simulink model "Simulation_model_full"  (R2021a)
settings: Solver=ode23t  StartTime=0.0  StopTime=6  FixedStep=T  RelTol=1e-3
values from neighbouring files (symbols this model uses):
  C_dc = Cb*c_dc_pu    [parameters.m]
  C_f = Cb*c_f_pu    [parameters.m]
  f_SM = fb    (= 50)    [parameters.m]
  fb = 50    [parameters.m]
  ff_SM = 0.01322    [parameters.m]
  Ib = 2/3*Sb/Vb    [parameters.m]
  Ib_dc = Sb/Vb_dc    [parameters.m]
  ic_SM = 0.8    [parameters.m]
  K_ad = 1.5    [parameters.m]
  K_ffv = 0    [parameters.m]
  K_ic = K_pc/T_1    [parameters.m]
  K_idc = K_pdc/T_idc    (= 250)    [parameters.m]
  K_iPLL = a^2*T_fPLL    (= 0.09)    [parameters.m]
  K_iv = K_pv/T_iv    (= 92.0050761421)    [parameters.m]
  K_iv_SM = K_pv_SM/T_iv_SM    (= 70)    [parameters.m]
  K_omega = 20    [parameters.m]
  K_omega_SM = 40    [parameters.m]
  K_pc = l_f_pu/(4*pi*fb*T_sum)    (= 1.27323954474)    [parameters.m]
  K_pdc = 25    [parameters.m]
  K_pPLL = 1/(a*2*pi*T_fPLL)    (= 5.30516476973)    [parameters.m]
  K_pv = 0.29    [parameters.m]
  K_pv_SM = 35    [parameters.m]
  K_vco = 2*pi    (= 6.28318530718)    [parameters.m]
  Kd = 40    [parameters.m]
  Kq = 0.1    [parameters.m]
  Kq_SM = 0.1    [parameters.m]
  L_f = Lb*l_f_pu    [parameters.m]
  l_f_pu = 0.08    [parameters.m]
  lfd_SM = 0.531    [parameters.m]
  llkd = 2.655    [parameters.m]
  llkq1 = 0.2408    [parameters.m]
  lls_SM = 0.08    [parameters.m]
  lmd_SM = 2.81    [parameters.m]
  lmq_SM = 1.64    [parameters.m]
  omega_ad = 50    [parameters.m]
  omega_b = 2*pi*fb    (= 314.159265359)    [parameters.m]
  omega_d = 5    [parameters.m]
  omega_qf = 200    [parameters.m]
  omega_qf_SM = 200    [parameters.m]
  omega_vf = 200    [parameters.m]
  p_h = 0.1    [parameters.m]
  pp_SM = 2    [parameters.m]
  R_lf = Rb*r_lf_pu    [parameters.m]
  rfd_SM = 0.004319    [parameters.m]
  rkd = 0.2343    [parameters.m]
  rkq1 = 0.03365    [parameters.m]
  rs_SM = 0.01524    [parameters.m]
  S_SM = Sb    (= 1000000)    [parameters.m]
  Sb = 1e6    (= 1000000)    [parameters.m]
  T = 1e-4    (= 0.0001)    [parameters.m]
  T_fPLL = 10e-3    (= 0.01)    [parameters.m]
  T_gt_SM = 0.5    [parameters.m]
  Ta = 4    [parameters.m]
  V_dc_bat = 1200    [parameters.m]
  v_dc_ref = 1    [parameters.m]
  V_SM = V    (= 690)    [parameters.m]
  Vb = V*sqrt(2)/sqrt(3)    [parameters.m]
  Vb_dc = Vb*2    [parameters.m]
undefined symbols (not defined in the file or in its folder): D1, Delta
libraries: simulink_extras x36, spsDiodeLib x24, spsThreePhaseVIMeasurementLib x16, spsThreePhaseSeriesRLCBranchLib x14, spsPower3phInstantaneousLib x8, spsVoltageMeasurementLib x5, spsControlledCurrentSourceLib x4, spsUniversalBridgeLib x4, spsParallelRLCBranchLib x2, spsSeriesRLCBranchLib x2, spsSynchronousMachinepuFundamentalLib x2, spsThreePhaseParallelRLCLoadLib x2
(part 2 of 3)

== system Simulation_model_full/Automatic Voltage Regulator SM A ==
  v_hat* : Inport
  v_hat_o : Inport  Port=2
  q* : Inport  Port=3
  qo : Inport  Port=4
  Gain15 : Gain  Gain=K_iv_SM
  Gain2 : Gain  Gain=Kq_SM
  Gain8 : Gain  Gain=K_pv_SM
  Integrator : Integrator
  Sum1 : Sum  Inputs=-++
  Sum2 : Sum  Inputs=|+-
  Sum9 : Sum  Inputs=|++
  Transfer Fcn (with initial outputs) : simulink_extras/Additional Linear/Transfer Fcn (with initial outputs)  N=[omega_qf_SM]  D="[1  omega_qf_SM]"  Y0=0  U0=0
  v_hat_e : Outport
  wires:
  Integrator/1 -> Sum9/2
  Sum1/1 -> Gain15/1, Gain8/1
  Gain15/1 -> Integrator/1
  Gain8/1 -> Sum9/1
  q*/1 -> Sum2/1
  qo/1 -> Transfer Fcn (with initial outputs)/1
  Transfer Fcn (with initial outputs)/1 -> Sum2/2
  Sum2/1 -> Gain2/1
  v_hat*/1 -> Sum1/2
  Gain2/1 -> Sum1/3
  Sum9/1 -> v_hat_e/1
  v_hat_o/1 -> Sum1/1

== system Simulation_model_full/Automatic Voltage Regulator SM B ==
  v_hat* : Inport
  v_hat_o : Inport  Port=2
  q* : Inport  Port=3
  qo : Inport  Port=4
  Gain15 : Gain  Gain=K_iv_SM
  Gain2 : Gain  Gain=Kq_SM
  Gain8 : Gain  Gain=K_pv_SM
  Integrator : Integrator
  Sum1 : Sum  Inputs=-++
  Sum2 : Sum  Inputs=|+-
  Sum9 : Sum  Inputs=|++
  Transfer Fcn (with initial outputs) : simulink_extras/Additional Linear/Transfer Fcn (with initial outputs)  N=[omega_qf_SM]  D="[1  omega_qf_SM]"  Y0=0  U0=0
  v_hat_e : Outport
  wires:
  Integrator/1 -> Sum9/2
  Sum1/1 -> Gain15/1, Gain8/1
  Gain15/1 -> Integrator/1
  Gain8/1 -> Sum9/1
  q*/1 -> Sum2/1
  qo/1 -> Transfer Fcn (with initial outputs)/1
  Transfer Fcn (with initial outputs)/1 -> Sum2/2
  Sum2/1 -> Gain2/1
  v_hat*/1 -> Sum1/2
  Gain2/1 -> Sum1/3
  Sum9/1 -> v_hat_e/1
  v_hat_o/1 -> Sum1/1

== system Simulation_model_full/Diesel Generator Governor Model SM A ==
  p*_sm : Inport
  omega_sm* : Inport  Port=2
  omega_sm : Inport  Port=3
  Sum1 : Sum  Inputs=++|
  Sum2 : Sum  Inputs=|+-
  Transfer Fcn (with initial outputs)2 : simulink_extras/Additional Linear/Transfer Fcn (with initial outputs)  N=[1]  D=[T_gt_SM 1]  Y0=0  U0=0
  "k_omega, sm" : Gain  Gain=K_omega_SM
  tau_dg : Outport
  wires:
  omega_sm*/1 -> Sum2/1
  omega_sm/1 -> Sum2/2
  Sum2/1 -> "k_omega, sm"/1
  "k_omega, sm"/1 -> Sum1/2
  p*_sm/1 -> Sum1/1
  Sum1/1 -> Transfer Fcn (with initial outputs)2/1
  Transfer Fcn (with initial outputs)2/1 -> tau_dg/1

== system Simulation_model_full/Diesel Generator Governor Model SM B ==
  p*_sm : Inport
  omega_sm* : Inport  Port=2
  omega_sm : Inport  Port=3
  Sum1 : Sum  Inputs=++|
  Sum2 : Sum  Inputs=|+-
  Transfer Fcn (with initial outputs)2 : simulink_extras/Additional Linear/Transfer Fcn (with initial outputs)  N=[1]  D=[T_gt_SM 1]  Y0=0  U0=0
  "k_omega, sm" : Gain  Gain=K_omega_SM
  tau_dg : Outport
  wires:
  omega_sm*/1 -> Sum2/1
  omega_sm/1 -> Sum2/2
  Sum2/1 -> "k_omega, sm"/1
  "k_omega, sm"/1 -> Sum1/2
  p*_sm/1 -> Sum1/1
  Sum1/1 -> Transfer Fcn (with initial outputs)2/1
  Transfer Fcn (with initial outputs)2/1 -> tau_dg/1

== system Simulation_model_full/P to I VSC A ==
  p_load : Inport
  v_dc : Inport  Port=2
  Divide : Product  Inputs=*/
  Saturation : Saturate  UpperLimit=1.5  LowerLimit=0.5
  Transfer Fcn (with initial outputs) : simulink_extras/Additional Linear/Transfer Fcn (with initial outputs)  N=[200]  D="[1  200]"  Y0=1  U0=1
  i_dc : Outport
  Out2 : Outport  Port=2
  wires:
  Divide/1 -> i_dc/1
  v_dc/1 -> Saturation/1
  Saturation/1 -> Transfer Fcn (with initial outputs)/1
  p_load/1 -> Divide/1
  Transfer Fcn (with initial outputs)/1 -> Divide/2

== system Simulation_model_full/P to I VSC B ==
  p_load : Inport
  v_dc : Inport  Port=2
  Divide : Product  Inputs=*/
  Saturation : Saturate  UpperLimit=1.5  LowerLimit=0.5
  Transfer Fcn (with initial outputs) : simulink_extras/Additional Linear/Transfer Fcn (with initial outputs)  N=[200]  D="[1  200]"  Y0=1  U0=1
  i_dc : Outport
  wires:
  Divide/1 -> i_dc/1
  v_dc/1 -> Saturation/1
  Saturation/1 -> Transfer Fcn (with initial outputs)/1
  p_load/1 -> Divide/1
  Transfer Fcn (with initial outputs)/1 -> Divide/2

== system Simulation_model_full/P to I 12puls A ==
  p* : Inport
  v_dc : Inport  Port=2
  Divide : Product  Inputs=*/
  Saturation : Saturate  UpperLimit=1.5  LowerLimit=0.5
  Transfer Fcn (with initial outputs) : simulink_extras/Additional Linear/Transfer Fcn (with initial outputs)  N=[200]  D="[1  200]"  Y0=1  U0=1
  i_dc : Outport
  wires:
  Divide/1 -> i_dc/1
  v_dc/1 -> Saturation/1
  Saturation/1 -> Transfer Fcn (with initial outputs)/1
  p*/1 -> Divide/1
  Transfer Fcn (with initial outputs)/1 -> Divide/2

== system Simulation_model_full/P to I 12puls B ==
  p* : Inport
  v_dc : Inport  Port=2
  Divide : Product  Inputs=*/
  Saturation : Saturate  UpperLimit=1.5  LowerLimit=0.5
  Transfer Fcn (with initial outputs) : simulink_extras/Additional Linear/Transfer Fcn (with initial outputs)  N=[200]  D="[1  200]"  Y0=1  U0=1
  i_dc : Outport
  wires:
  Divide/1 -> i_dc/1
  v_dc/1 -> Saturation/1
  Saturation/1 -> Transfer Fcn (with initial outputs)/1
  p*/1 -> Divide/1
  Transfer Fcn (with initial outputs)/1 -> Divide/2

== system Simulation_model_full/PLL grid ==
  Vo : Inport
  Atan2 : Trigonometry  Operator=atan2  OutputSignalType=real
  Constant1 : Constant  Value=fb
  Demux : Demux  Outputs=3
  Gain : Gain  Gain=K_vco
  Gain12 : Gain  Gain=1/omega_b
  Gain17 : Gain  Gain=K_iPLL
  Gain18 : Gain  Gain=K_pPLL
  Integrator2 : Integrator
  Park : MATLAB Function  TreatAsAtomicUnit=on
  Sum1 : Sum  Inputs=++|
  Sum10 : Sum  Inputs=++|
  Terminator : Terminator
  Transfer Fcn (with initial outputs)1 : simulink_extras/Additional Linear/Transfer Fcn (with initial outputs)  N=[1]  D=[T_fPLL, 1]  Y0=0  U0=0
  Transfer Fcn (with initial outputs)3 : simulink_extras/Additional Linear/Transfer Fcn (with initial outputs)  N=[1]  D=[T_fPLL, 1]  Y0=1  U0=1
  VCO : Integrator  WrapState=on  WrappedStateUpperValue=2*pi  WrappedStateLowerValue=0
  abs vhat_f VSM : MATLAB Function  TreatAsAtomicUnit=on
  omega : Outport
  v_hat : Outport  Port=2
  wires:
  Transfer Fcn (with initial outputs)1/1 -> Atan2/1, abs vhat_f VSM/2(vq)
  Transfer Fcn (with initial outputs)3/1 -> Atan2/2, abs vhat_f VSM/1(vd)
  VCO/1 -> Park/1(theta)
  Sum1/1 -> Gain/1
  Gain/1 -> Gain12/1, VCO/1
  Constant1/1 -> Sum1/1
  Park/1(dq0) -> Demux/1
  Sum10/1 -> Sum1/2
  Atan2/1 -> Gain18/1, Gain17/1
  Demux/1 -> Transfer Fcn (with initial outputs)3/1
  Demux/2 -> Transfer Fcn (with initial outputs)1/1
  Vo/1 -> Park/2(abc)
  Gain18/1 -> Sum10/2
  Integrator2/1 -> Sum10/1
  Gain17/1 -> Integrator2/1
  Gain12/1 -> omega/1
  Demux/3 -> Terminator/1
  abs vhat_f VSM/1(v_abs) -> v_hat/1

== system Simulation_model_full/PLL grid1 ==
  Vo : Inport
  Atan2 : Trigonometry  Operator=atan2  OutputSignalType=real
  Constant1 : Constant  Value=fb
  Demux : Demux  Outputs=3
  Gain : Gain  Gain=K_vco
  Gain12 : Gain  Gain=1/omega_b
  Gain17 : Gain  Gain=K_iPLL
  Gain18 : Gain  Gain=K_pPLL
  Integrator2 : Integrator
  Park : MATLAB Function  TreatAsAtomicUnit=on
  Sum1 : Sum  Inputs=++|
  Sum10 : Sum  Inputs=++|
  Terminator : Terminator
  Transfer Fcn (with initial outputs)1 : simulink_extras/Additional Linear/Transfer Fcn (with initial outputs)  N=[1]  D=[T_fPLL, 1]  Y0=0  U0=0
  Transfer Fcn (with initial outputs)3 : simulink_extras/Additional Linear/Transfer Fcn (with initial outputs)  N=[1]  D=[T_fPLL, 1]  Y0=1  U0=1
  VCO : Integrator  WrapState=on  WrappedStateUpperValue=2*pi  WrappedStateLowerValue=0
  abs vhat_f VSM : MATLAB Function  TreatAsAtomicUnit=on
  omega : Outport
  v_hat : Outport  Port=2
  wires:
  Transfer Fcn (with initial outputs)1/1 -> Atan2/1, abs vhat_f VSM/2(vq)
  Transfer Fcn (with initial outputs)3/1 -> Atan2/2, abs vhat_f VSM/1(vd)
  VCO/1 -> Park/1(theta)
  Sum1/1 -> Gain/1
  Gain/1 -> Gain12/1, VCO/1
  Constant1/1 -> Sum1/1
  Park/1(dq0) -> Demux/1
  Sum10/1 -> Sum1/2
  Atan2/1 -> Gain18/1, Gain17/1
  Demux/1 -> Transfer Fcn (with initial outputs)3/1
  Demux/2 -> Transfer Fcn (with initial outputs)1/1
  Vo/1 -> Park/2(abc)
  Gain18/1 -> Sum10/2
  Integrator2/1 -> Sum10/1
  Gain17/1 -> Integrator2/1
  Gain12/1 -> omega/1
  Demux/3 -> Terminator/1
  abs vhat_f VSM/1(v_abs) -> v_hat/1

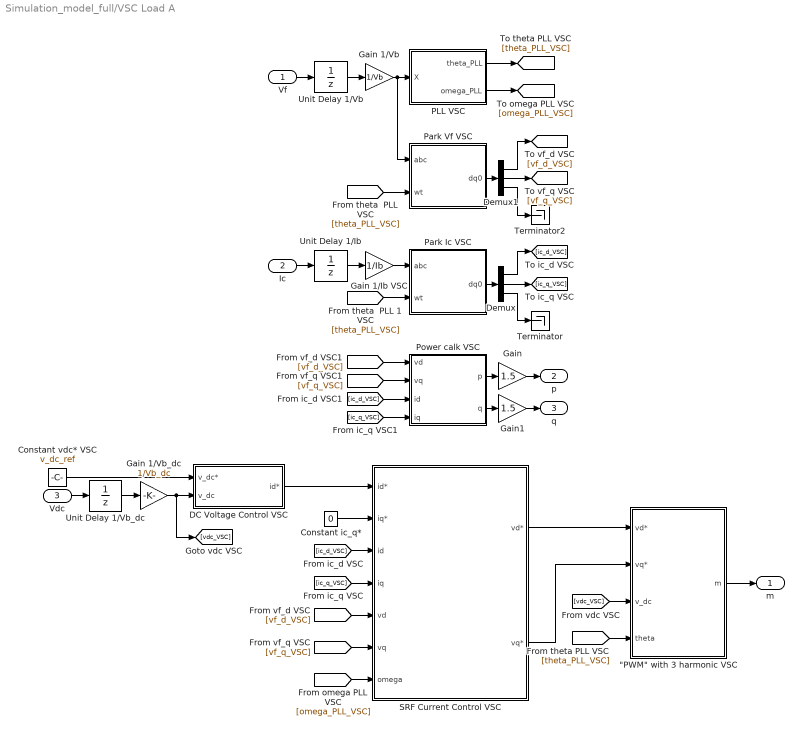
== system Simulation_model_full/VSC Load A ==
  Vf : Inport
  Ic : Inport  Port=2
  Vdc : Inport  Port=3
  "\"PWM\" with 3 harmonic VSC" : Subsystem
  Constant ic_q* : Constant  Value=0
  Constant vdc* VSC : Constant  Value=v_dc_ref
  DC Voltage Control VSC : Subsystem
  Demux : Demux  Outputs=3
  Demux1 : Demux  Outputs=3
  Gain : Gain  Gain=1.5
  Gain 1/Ib VSC : Gain  Gain=1/Ib
  Gain 1/Vb : Gain  Gain=1/Vb
  Gain 1/Vb_dc : Gain  Gain=1/Vb_dc
  Gain1 : Gain  Gain=1.5
  PLL VSC : Subsystem
  Park Ic VSC : MATLAB Function  TreatAsAtomicUnit=on
  Park Vf VSC : MATLAB Function  TreatAsAtomicUnit=on
  Power calk VSC : MATLAB Function  TreatAsAtomicUnit=on
  SRF Current Control VSC : Subsystem
  Terminator : Terminator
  Terminator2 : Terminator
  Unit Delay 1/Ib : UnitDelay  SampleTime=-1  HasFrameUpgradeWarning=on
  Unit Delay 1/Vb : UnitDelay  SampleTime=-1  HasFrameUpgradeWarning=on
  "Unit Delay 1/Vb_dc " : UnitDelay  InitialCondition=Vb_dc  SampleTime=-1  HasFrameUpgradeWarning=on
  m : Outport
  p : Outport  Port=2
  q : Outport  Port=3
  wires:
  Constant vdc* VSC/1 -> DC Voltage Control VSC/1(v_dc*)
  [theta_PLL_VSC] -> Park Ic VSC/2(wt)
  Gain 1/Ib VSC/1 -> Park Ic VSC/1(abc)
  Vf/1 -> Unit Delay 1/Vb/1
  Gain 1/Vb_dc/1 -> [vdc_VSC], DC Voltage Control VSC/2(v_dc)
  [ic_d_VSC] -> Power calk VSC/3(id)
  Gain 1/Vb/1 -> Park Vf VSC/1(abc), PLL VSC/1(X)
  Demux1/2 -> [vf_q_VSC]
  [omega_PLL_VSC] -> SRF Current Control VSC/7(omega)
  Demux1/3 -> Terminator2/1
  [vf_d_VSC] -> Power calk VSC/1(vd)
  Park Ic VSC/1(dq0) -> Demux/1
  [ic_q_VSC] -> Power calk VSC/4(iq)
  PLL VSC/2(omega_PLL) -> [omega_PLL_VSC]
  PLL VSC/1(theta_PLL) -> [theta_PLL_VSC]
  SRF Current Control VSC/2(vq*) -> "\"PWM\" with 3 harmonic VSC"/2(vq*)
  [vf_q_VSC] -> SRF Current Control VSC/6(vq)
  Unit Delay 1/Ib/1 -> Gain 1/Ib VSC/1
  Park Vf VSC/1(dq0) -> Demux1/1
  [vf_q_VSC] -> Power calk VSC/2(vq)
  Demux1/1 -> [vf_d_VSC]
  [theta_PLL_VSC] -> "\"PWM\" with 3 harmonic VSC"/4(theta)
  Demux/1 -> [ic_d_VSC]
  Gain/1 -> p/1
  Unit Delay 1/Vb/1 -> Gain 1/Vb/1
  [theta_PLL_VSC] -> Park Vf VSC/2(wt)
  [ic_d_VSC] -> SRF Current Control VSC/3(id)
  [ic_q_VSC] -> SRF Current Control VSC/4(iq)
  Demux/2 -> [ic_q_VSC]
  DC Voltage Control VSC/1(id*) -> SRF Current Control VSC/1(id*)
  SRF Current Control VSC/1(vd*) -> "\"PWM\" with 3 harmonic VSC"/1(vd*)
  Demux/3 -> Terminator/1
  [vdc_VSC] -> "\"PWM\" with 3 harmonic VSC"/3(v_dc)
  Constant ic_q*/1 -> SRF Current Control VSC/2(iq*)
  "Unit Delay 1/Vb_dc "/1 -> Gain 1/Vb_dc/1
  [vf_d_VSC] -> SRF Current Control VSC/5(vd)
  Ic/1 -> Unit Delay 1/Ib/1
  Vdc/1 -> "Unit Delay 1/Vb_dc "/1
  "\"PWM\" with 3 harmonic VSC"/1(m) -> m/1
  Power calk VSC/1(p) -> Gain/1
  Power calk VSC/2(q) -> Gain1/1
  Gain1/1 -> q/1

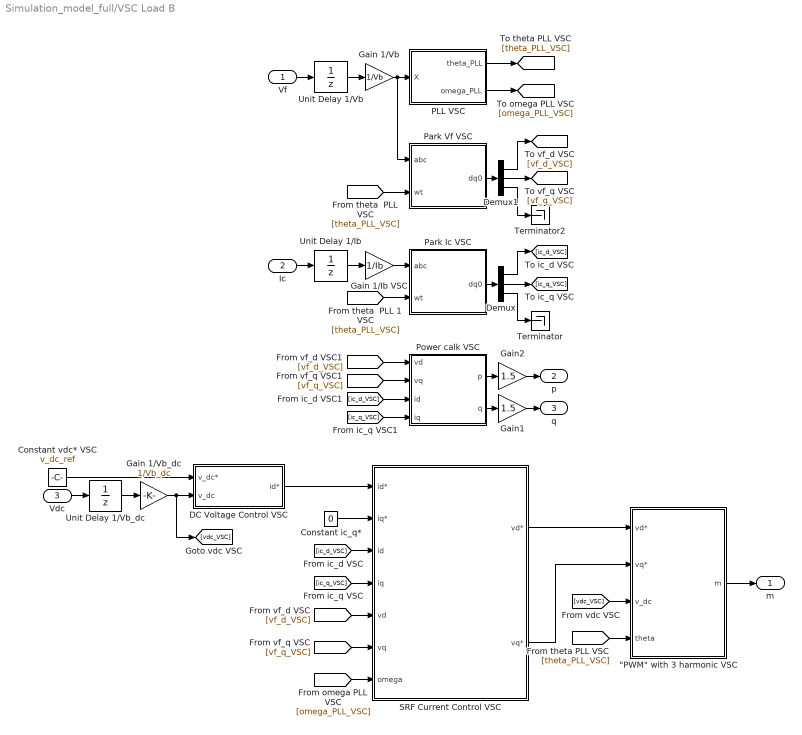
== system Simulation_model_full/VSC Load B ==
  Vf : Inport
  Ic : Inport  Port=2
  Vdc : Inport  Port=3
  "\"PWM\" with 3 harmonic VSC" : Subsystem
  Constant ic_q* : Constant  Value=0
  Constant vdc* VSC : Constant  Value=v_dc_ref
  DC Voltage Control VSC : Subsystem
  Demux : Demux  Outputs=3
  Demux1 : Demux  Outputs=3
  Gain 1/Ib VSC : Gain  Gain=1/Ib
  Gain 1/Vb : Gain  Gain=1/Vb
  Gain 1/Vb_dc : Gain  Gain=1/Vb_dc
  Gain1 : Gain  Gain=1.5
  Gain2 : Gain  Gain=1.5
  PLL VSC : Subsystem
  Park Ic VSC : MATLAB Function  TreatAsAtomicUnit=on
  Park Vf VSC : MATLAB Function  TreatAsAtomicUnit=on
  Power calk VSC : MATLAB Function  TreatAsAtomicUnit=on
  SRF Current Control VSC : Subsystem
  Terminator : Terminator
  Terminator2 : Terminator
  Unit Delay 1/Ib : UnitDelay  SampleTime=-1  HasFrameUpgradeWarning=on
  Unit Delay 1/Vb : UnitDelay  SampleTime=-1  HasFrameUpgradeWarning=on
  "Unit Delay 1/Vb_dc " : UnitDelay  InitialCondition=Vb_dc  SampleTime=-1  HasFrameUpgradeWarning=on
  m : Outport
  p : Outport  Port=2
  q : Outport  Port=3
  wires:
  Constant vdc* VSC/1 -> DC Voltage Control VSC/1(v_dc*)
  [theta_PLL_VSC] -> Park Ic VSC/2(wt)
  Gain 1/Ib VSC/1 -> Park Ic VSC/1(abc)
  Vf/1 -> Unit Delay 1/Vb/1
  Gain 1/Vb_dc/1 -> [vdc_VSC], DC Voltage Control VSC/2(v_dc)
  [ic_d_VSC] -> Power calk VSC/3(id)
  Gain 1/Vb/1 -> Park Vf VSC/1(abc), PLL VSC/1(X)
  Demux1/2 -> [vf_q_VSC]
  [omega_PLL_VSC] -> SRF Current Control VSC/7(omega)
  Demux1/3 -> Terminator2/1
  [vf_d_VSC] -> Power calk VSC/1(vd)
  Park Ic VSC/1(dq0) -> Demux/1
  [ic_q_VSC] -> Power calk VSC/4(iq)
  PLL VSC/2(omega_PLL) -> [omega_PLL_VSC]
  PLL VSC/1(theta_PLL) -> [theta_PLL_VSC]
  SRF Current Control VSC/2(vq*) -> "\"PWM\" with 3 harmonic VSC"/2(vq*)
  [vf_q_VSC] -> SRF Current Control VSC/6(vq)
  Unit Delay 1/Ib/1 -> Gain 1/Ib VSC/1
  Park Vf VSC/1(dq0) -> Demux1/1
  [vf_q_VSC] -> Power calk VSC/2(vq)
  Demux1/1 -> [vf_d_VSC]
  [theta_PLL_VSC] -> "\"PWM\" with 3 harmonic VSC"/4(theta)
  Demux/1 -> [ic_d_VSC]
  Unit Delay 1/Vb/1 -> Gain 1/Vb/1
  [theta_PLL_VSC] -> Park Vf VSC/2(wt)
  [ic_d_VSC] -> SRF Current Control VSC/3(id)
  [ic_q_VSC] -> SRF Current Control VSC/4(iq)
  Demux/2 -> [ic_q_VSC]
  DC Voltage Control VSC/1(id*) -> SRF Current Control VSC/1(id*)
  SRF Current Control VSC/1(vd*) -> "\"PWM\" with 3 harmonic VSC"/1(vd*)
  Demux/3 -> Terminator/1
  [vdc_VSC] -> "\"PWM\" with 3 harmonic VSC"/3(v_dc)
  Constant ic_q*/1 -> SRF Current Control VSC/2(iq*)
  "Unit Delay 1/Vb_dc "/1 -> Gain 1/Vb_dc/1
  [vf_d_VSC] -> SRF Current Control VSC/5(vd)
  Ic/1 -> Unit Delay 1/Ib/1
  Vdc/1 -> "Unit Delay 1/Vb_dc "/1
  "\"PWM\" with 3 harmonic VSC"/1(m) -> m/1
  Power calk VSC/1(p) -> Gain2/1
  Gain2/1 -> p/1
  Power calk VSC/2(q) -> Gain1/1
  Gain1/1 -> q/1

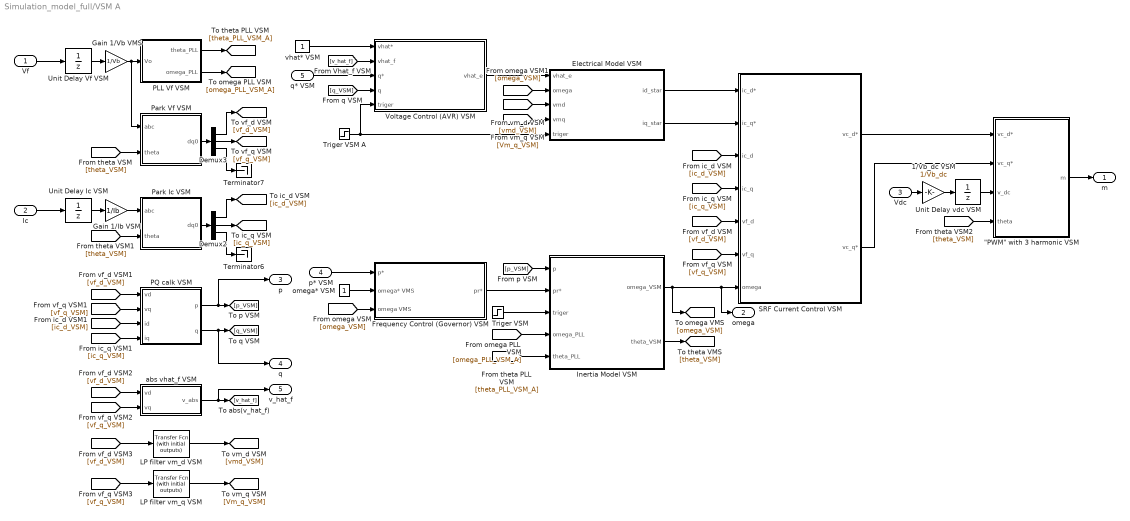
== system Simulation_model_full/VSM A ==
  Vf : Inport
  Ic : Inport  Port=2
  Vdc : Inport  Port=3
  p* VSM : Inport  Port=4
  q* VSM : Inport  Port=5
  "\"PWM\" with 3 harmonic VSM" : Subsystem
  1/Vb_dc VSM : Gain  Gain=1/Vb_dc
  Demux2 : Demux  Outputs=3
  Demux3 : Demux  Outputs=3
  Electrical Model VSM : MATLAB Function  TreatAsAtomicUnit=on
  Frequency Control (Governor) VSM : Subsystem
  Gain 1/Ib VSM : Gain  Gain=1/Ib
  Gain 1/Vb VMS : Gain  Gain=1/Vb
  Inertia Model VSM : Subsystem
  LP filter vm_d VSM : simulink_extras/Additional Linear/Transfer Fcn (with initial outputs)  N=[omega_vf]  D="[1  omega_vf]"  Y0=1  U0=1
  LP filter vm_q VSM : simulink_extras/Additional Linear/Transfer Fcn (with initial outputs)  N=[omega_vf]  D="[1  omega_vf]"  Y0=0  U0=0
  PLL Vf VSM : Subsystem
  PQ calk VSM : MATLAB Function  TreatAsAtomicUnit=on
  Park Ic VSM : MATLAB Function  TreatAsAtomicUnit=on
  Park Vf VSM : MATLAB Function  TreatAsAtomicUnit=on
  SRF Current Control VSM : Subsystem
  Terminator6 : Terminator
  Terminator7 : Terminator
  Triger VSM : Step  Time=0  Before=1  After=0  SampleTime=0
  Triger VSM A : Step  Time=0  Before=1  After=0  SampleTime=0
  Unit Delay Ic VSM : UnitDelay  SampleTime=-1  HasFrameUpgradeWarning=on
  Unit Delay Vf VSM : UnitDelay  SampleTime=-1  HasFrameUpgradeWarning=on
  Unit Delay vdc VSM : UnitDelay  InitialCondition=1  SampleTime=-1  HasFrameUpgradeWarning=on
  Voltage Control (AVR) VSM : Subsystem
  abs vhat_f VSM : MATLAB Function  TreatAsAtomicUnit=on
  omega* VSM : Constant
  vhat* VSM : Constant
  m : Outport
  omega : Outport  Port=2
  p : Outport  Port=3
  q : Outport  Port=4
  v_hat_f : Outport  Port=5
  wires:
  [theta_VSM] -> Park Vf VSM/2(theta)
  [theta_VSM] -> "\"PWM\" with 3 harmonic VSM"/4(theta)
  [vf_q_VSM] -> SRF Current Control VSM/6(vf_q)
  Demux3/1 -> [vf_d_VSM]
  [q_VSM] -> Voltage Control (AVR) VSM/4(q)
  [vf_d_VSM] -> PQ calk VSM/1(vd)
  SRF Current Control VSM/2(vc_q*) -> "\"PWM\" with 3 harmonic VSM"/2(vc_q*)
  Park Ic VSM/1(dq0) -> Demux2/1
  Vdc/1 -> 1/Vb_dc VSM/1
  Unit Delay vdc VSM/1 -> "\"PWM\" with 3 harmonic VSM"/3(v_dc)
  Vf/1 -> Unit Delay Vf VSM/1
  omega* VSM/1 -> Frequency Control (Governor) VSM/2(omega* VMS)
  [theta_VSM] -> Park Ic VSM/2(theta)
  Demux2/2 -> [ic_q_VSM]
  [omega_VSM] -> Frequency Control (Governor) VSM/3(omega VMS)
  LP filter vm_d VSM/1 -> [vmd_VSM]
  [ic_d_VSM] -> PQ calk VSM/3(id)
  [vf_d_VSM] -> abs vhat_f VSM/1(vd)
  LP filter vm_q VSM/1 -> [Vm_q_VSM]
  Demux3/3 -> Terminator7/1
  1/Vb_dc VSM/1 -> Unit Delay vdc VSM/1
  Inertia Model VSM/2(theta_VSM) -> [theta_VSM]
  [ic_q_VSM] -> PQ calk VSM/4(iq)
  [vf_q_VSM] -> LP filter vm_q VSM/1
  Electrical Model VSM/1(id_star) -> SRF Current Control VSM/1(ic_d*)
  [vmd_VSM] -> Electrical Model VSM/3(vmd)
  [vf_q_VSM] -> abs vhat_f VSM/2(vq)
  "\"PWM\" with 3 harmonic VSM"/1(m) -> m/1
  [p_VSM] -> Inertia Model VSM/1(p)
  [v_hat_f] -> Voltage Control (AVR) VSM/2(vhat_f)
  [ic_q_VSM] -> SRF Current Control VSM/4(ic_q)
  Gain 1/Vb VMS/1 -> Park Vf VSM/1(abc), PLL Vf VSM/1(Vo)
  PLL Vf VSM/2(omega_PLL) -> [omega_PLL_VSM_A]
  p* VSM/1 -> Frequency Control (Governor) VSM/1(p*)
  [omega_PLL_VSM_A] -> Inertia Model VSM/4(omega_PLL)
  PLL Vf VSM/1(theta_PLL) -> [theta_PLL_VSM_A]
  Frequency Control (Governor) VSM/1(pr*) -> Inertia Model VSM/2(pr*)
  [theta_PLL_VSM_A] -> Inertia Model VSM/5(theta_PLL)
  Unit Delay Ic VSM/1 -> Gain 1/Ib VSM/1
  Electrical Model VSM/2(iq_star) -> SRF Current Control VSM/2(ic_q*)
  Triger VSM A/1 -> Voltage Control (AVR) VSM/5(triger), Electrical Model VSM/5(triger)
  q* VSM/1 -> Voltage Control (AVR) VSM/3(q*)
  Demux2/1 -> [ic_d_VSM]
  Voltage Control (AVR) VSM/1(vhat_e) -> Electrical Model VSM/1(vhat_e)
  [omega_VSM] -> Electrical Model VSM/2(omega)
  vhat* VSM/1 -> Voltage Control (AVR) VSM/1(vhat*)
  SRF Current Control VSM/1(vc_d*) -> "\"PWM\" with 3 harmonic VSM"/1(vc_d*)
  [vf_d_VSM] -> LP filter vm_d VSM/1
  Triger VSM/1 -> Inertia Model VSM/3(triger)
  Demux2/3 -> Terminator6/1
  [Vm_q_VSM] -> Electrical Model VSM/4(vmq)
  [vf_d_VSM] -> SRF Current Control VSM/5(vf_d)
  Inertia Model VSM/1(omega_VSM) -> [omega_VSM], SRF Current Control VSM/7(omega), omega/1
  [ic_d_VSM] -> SRF Current Control VSM/3(ic_d)
  Gain 1/Ib VSM/1 -> Park Ic VSM/1(abc)
  Demux3/2 -> [vf_q_VSM]
  [vf_q_VSM] -> PQ calk VSM/2(vq)
  Unit Delay Vf VSM/1 -> Gain 1/Vb VMS/1
  Park Vf VSM/1(dq0) -> Demux3/1
  abs vhat_f VSM/1(v_abs) -> v_hat_f/1, [v_hat_f]
  Ic/1 -> Unit Delay Ic VSM/1
  PQ calk VSM/1(p) -> p/1, [p_VSM]
  PQ calk VSM/2(q) -> q/1, [q_VSM]

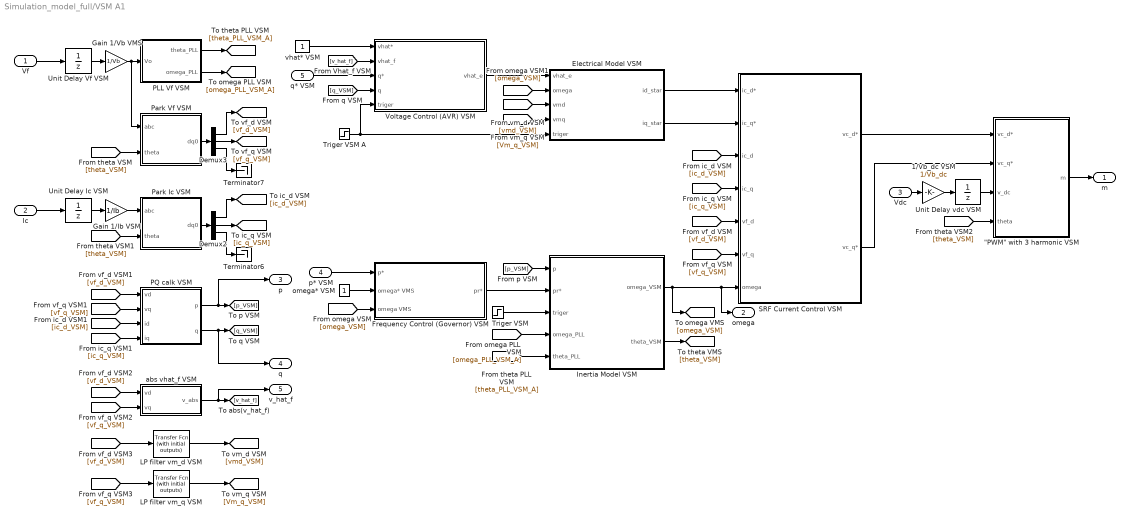
== system Simulation_model_full/VSM A1 ==
  Vf : Inport
  Ic : Inport  Port=2
  Vdc : Inport  Port=3
  p* VSM : Inport  Port=4
  q* VSM : Inport  Port=5
  "\"PWM\" with 3 harmonic VSM" : Subsystem
  1/Vb_dc VSM : Gain  Gain=1/Vb_dc
  Demux2 : Demux  Outputs=3
  Demux3 : Demux  Outputs=3
  Electrical Model VSM : MATLAB Function  TreatAsAtomicUnit=on
  Frequency Control (Governor) VSM : Subsystem
  Gain 1/Ib VSM : Gain  Gain=1/Ib
  Gain 1/Vb VMS : Gain  Gain=1/Vb
  Inertia Model VSM : Subsystem
  LP filter vm_d VSM : simulink_extras/Additional Linear/Transfer Fcn (with initial outputs)  N=[omega_vf]  D="[1  omega_vf]"  Y0=1  U0=1
  LP filter vm_q VSM : simulink_extras/Additional Linear/Transfer Fcn (with initial outputs)  N=[omega_vf]  D="[1  omega_vf]"  Y0=0  U0=0
  PLL Vf VSM : Subsystem
  PQ calk VSM : MATLAB Function  TreatAsAtomicUnit=on
  Park Ic VSM : MATLAB Function  TreatAsAtomicUnit=on
  Park Vf VSM : MATLAB Function  TreatAsAtomicUnit=on
  SRF Current Control VSM : Subsystem
  Terminator6 : Terminator
  Terminator7 : Terminator
  Triger VSM : Step  Time=0  Before=1  After=0  SampleTime=0
  Triger VSM A : Step  Time=0  Before=1  After=0  SampleTime=0
  Unit Delay Ic VSM : UnitDelay  SampleTime=-1  HasFrameUpgradeWarning=on
  Unit Delay Vf VSM : UnitDelay  SampleTime=-1  HasFrameUpgradeWarning=on
  Unit Delay vdc VSM : UnitDelay  InitialCondition=1  SampleTime=-1  HasFrameUpgradeWarning=on
  Voltage Control (AVR) VSM : Subsystem
  abs vhat_f VSM : MATLAB Function  TreatAsAtomicUnit=on
  omega* VSM : Constant
  vhat* VSM : Constant
  m : Outport
  omega : Outport  Port=2
  p : Outport  Port=3
  q : Outport  Port=4
  v_hat_f : Outport  Port=5
  wires:
  [theta_VSM] -> Park Vf VSM/2(theta)
  [theta_VSM] -> "\"PWM\" with 3 harmonic VSM"/4(theta)
  [vf_q_VSM] -> SRF Current Control VSM/6(vf_q)
  Demux3/1 -> [vf_d_VSM]
  [q_VSM] -> Voltage Control (AVR) VSM/4(q)
  [vf_d_VSM] -> PQ calk VSM/1(vd)
  SRF Current Control VSM/2(vc_q*) -> "\"PWM\" with 3 harmonic VSM"/2(vc_q*)
  Park Ic VSM/1(dq0) -> Demux2/1
  Vdc/1 -> 1/Vb_dc VSM/1
  Unit Delay vdc VSM/1 -> "\"PWM\" with 3 harmonic VSM"/3(v_dc)
  Vf/1 -> Unit Delay Vf VSM/1
  omega* VSM/1 -> Frequency Control (Governor) VSM/2(omega* VMS)
  [theta_VSM] -> Park Ic VSM/2(theta)
  Demux2/2 -> [ic_q_VSM]
  [omega_VSM] -> Frequency Control (Governor) VSM/3(omega VMS)
  LP filter vm_d VSM/1 -> [vmd_VSM]
  [ic_d_VSM] -> PQ calk VSM/3(id)
  [vf_d_VSM] -> abs vhat_f VSM/1(vd)
  LP filter vm_q VSM/1 -> [Vm_q_VSM]
  Demux3/3 -> Terminator7/1
  1/Vb_dc VSM/1 -> Unit Delay vdc VSM/1
  Inertia Model VSM/2(theta_VSM) -> [theta_VSM]
  [ic_q_VSM] -> PQ calk VSM/4(iq)
  [vf_q_VSM] -> LP filter vm_q VSM/1
  Electrical Model VSM/1(id_star) -> SRF Current Control VSM/1(ic_d*)
  [vmd_VSM] -> Electrical Model VSM/3(vmd)
  [vf_q_VSM] -> abs vhat_f VSM/2(vq)
  "\"PWM\" with 3 harmonic VSM"/1(m) -> m/1
  [p_VSM] -> Inertia Model VSM/1(p)
  [v_hat_f] -> Voltage Control (AVR) VSM/2(vhat_f)
  [ic_q_VSM] -> SRF Current Control VSM/4(ic_q)
  Gain 1/Vb VMS/1 -> Park Vf VSM/1(abc), PLL Vf VSM/1(Vo)
  PLL Vf VSM/2(omega_PLL) -> [omega_PLL_VSM_A]
  p* VSM/1 -> Frequency Control (Governor) VSM/1(p*)
  [omega_PLL_VSM_A] -> Inertia Model VSM/4(omega_PLL)
  PLL Vf VSM/1(theta_PLL) -> [theta_PLL_VSM_A]
  Frequency Control (Governor) VSM/1(pr*) -> Inertia Model VSM/2(pr*)
  [theta_PLL_VSM_A] -> Inertia Model VSM/5(theta_PLL)
  Unit Delay Ic VSM/1 -> Gain 1/Ib VSM/1
  Electrical Model VSM/2(iq_star) -> SRF Current Control VSM/2(ic_q*)
  Triger VSM A/1 -> Voltage Control (AVR) VSM/5(triger), Electrical Model VSM/5(triger)
  q* VSM/1 -> Voltage Control (AVR) VSM/3(q*)
  Demux2/1 -> [ic_d_VSM]
  Voltage Control (AVR) VSM/1(vhat_e) -> Electrical Model VSM/1(vhat_e)
  [omega_VSM] -> Electrical Model VSM/2(omega)
  vhat* VSM/1 -> Voltage Control (AVR) VSM/1(vhat*)
  SRF Current Control VSM/1(vc_d*) -> "\"PWM\" with 3 harmonic VSM"/1(vc_d*)
  [vf_d_VSM] -> LP filter vm_d VSM/1
  Triger VSM/1 -> Inertia Model VSM/3(triger)
  Demux2/3 -> Terminator6/1
  [Vm_q_VSM] -> Electrical Model VSM/4(vmq)
  [vf_d_VSM] -> SRF Current Control VSM/5(vf_d)
  Inertia Model VSM/1(omega_VSM) -> [omega_VSM], SRF Current Control VSM/7(omega), omega/1
  [ic_d_VSM] -> SRF Current Control VSM/3(ic_d)
  Gain 1/Ib VSM/1 -> Park Ic VSM/1(abc)
  Demux3/2 -> [vf_q_VSM]
  [vf_q_VSM] -> PQ calk VSM/2(vq)
  Unit Delay Vf VSM/1 -> Gain 1/Vb VMS/1
  Park Vf VSM/1(dq0) -> Demux3/1
  abs vhat_f VSM/1(v_abs) -> v_hat_f/1, [v_hat_f]
  Ic/1 -> Unit Delay Ic VSM/1
  PQ calk VSM/1(p) -> p/1, [p_VSM]
  PQ calk VSM/2(q) -> q/1, [q_VSM]

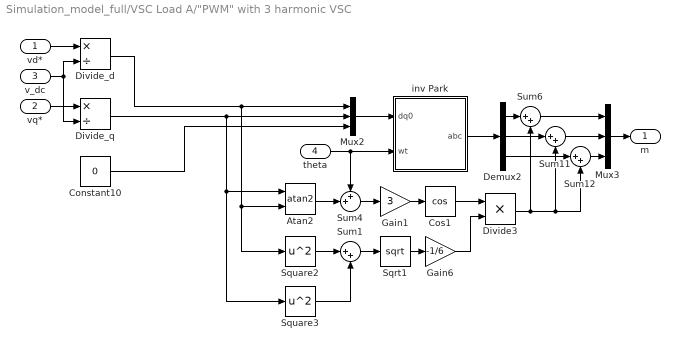
== system Simulation_model_full/VSC Load A/"PWM" with 3 harmonic VSC ==
  vd* : Inport
  vq* : Inport  Port=2
  v_dc : Inport  Port=3
  theta : Inport  Port=4
  Atan2 : Trigonometry  Operator=atan2
  Constant10 : Constant  Value=0
  Cos1 : Trigonometry  Operator=cos
  Demux2 : Demux  Outputs=3
  Divide3 : Product  Inputs=**
  Divide_d : Product  Inputs=*/
  Divide_q : Product  Inputs=*/
  Gain1 : Gain  Gain=3
  Gain6 : Gain  Gain=-1/6
  Mux2 : Mux  Inputs=3
  Mux3 : Mux  Inputs=3
  Sqrt1 : Sqrt  SaturateOnIntegerOverflow=on
  Square2 : Math  Operator=square  SaturateOnIntegerOverflow=on
  Square3 : Math  Operator=square  SaturateOnIntegerOverflow=on
  Sum{1,6,11..12} (4 alike) : Sum  Inputs=|++
  Sum4 : Sum  Inputs=++|
  inv Park : MATLAB Function  TreatAsAtomicUnit=on
  m : Outport
  wires:
  Constant10/1 -> Mux2/3
  Demux2/2 -> Sum11/1
  Sum4/1 -> Gain1/1
  Square2/1 -> Sum1/1
  Demux2/3 -> Sum12/1
  Divide3/1 -> Sum12/2, Sum11/2, Sum6/2
  Atan2/1 -> Sum4/2
  theta/1 -> Sum4/1, inv Park/2(wt)
  Gain6/1 -> Divide3/2
  Gain1/1 -> Cos1/1
  Sum12/1 -> Mux3/3
  Demux2/1 -> Sum6/1
  Sum6/1 -> Mux3/1
  Square3/1 -> Sum1/2
  Sum1/1 -> Sqrt1/1
  Cos1/1 -> Divide3/1
  Sum11/1 -> Mux3/2
  Sqrt1/1 -> Gain6/1
  Mux2/1 -> inv Park/1(dq0)
  vq*/1 -> Divide_q/1
  v_dc/1 -> Divide_d/2, Divide_q/2
  vd*/1 -> Divide_d/1
  Divide_d/1 -> Mux2/1, Atan2/2, Square2/1
  Divide_q/1 -> Square3/1, Atan2/1, Mux2/2
  Mux3/1 -> m/1
  inv Park/1(abc) -> Demux2/1

== system Simulation_model_full/VSC Load A/DC Voltage Control VSC ==
  v_dc* : Inport
  v_dc : Inport  Port=2
  Gain : Gain  Gain=-1
  Gain20 : Gain  Gain=K_idc
  Gain21 : Gain  Gain=K_pdc
  Integrator3 : Integrator
  Sum15 : Sum  Inputs=|++
  Sum16 : Sum  Inputs=|+-
  id* : Outport
  wires:
  Gain21/1 -> Sum15/1
  Sum16/1 -> Gain21/1, Gain20/1
  Integrator3/1 -> Sum15/2
  v_dc*/1 -> Sum16/1
  v_dc/1 -> Sum16/2
  Gain20/1 -> Integrator3/1
  Sum15/1 -> Gain/1
  Gain/1 -> id*/1

== system Simulation_model_full/VSC Load A/PLL VSC ==
  X : Inport
  Atan2 : Trigonometry  Operator=atan2  OutputSignalType=real
  Constant : Constant  Value=0
  Constant1 : Constant  Value=fb
  Demux : Demux  Outputs=3
  Gain : Gain  Gain=K_vco
  Gain12 : Gain  Gain=1/omega_b
  Gain17 : Gain  Gain=K_iPLL
  Gain18 : Gain  Gain=K_pPLL
  Integrator2 : Integrator
  Park : MATLAB Function  TreatAsAtomicUnit=on
  Sum : Sum  Inputs=|++
  Sum1 : Sum  Inputs=++|
  Sum10 : Sum  Inputs=++|
  Terminator : Terminator
  Transfer Fcn (with initial outputs)1 : simulink_extras/Additional Linear/Transfer Fcn (with initial outputs)  N=[1]  D=[T_fPLL, 1]  Y0=0  U0=0
  Transfer Fcn (with initial outputs)3 : simulink_extras/Additional Linear/Transfer Fcn (with initial outputs)  N=[1]  D=[T_fPLL, 1]  Y0=1  U0=1
  VCO : Integrator  WrapState=on  WrappedStateUpperValue=2*pi  WrappedStateLowerValue=0
  theta_PLL : Outport
  omega_PLL : Outport  Port=2
  wires:
  Transfer Fcn (with initial outputs)1/1 -> Atan2/1
  Transfer Fcn (with initial outputs)3/1 -> Atan2/2
  Constant/1 -> Sum/1
  VCO/1 -> theta_PLL/1, Park/1(wt)
  Sum1/1 -> Gain/1
  Gain/1 -> Gain12/1, VCO/1
  Constant1/1 -> Sum1/1
  Park/1(dq0) -> Demux/1
  Atan2/1 -> Sum/2
  Sum10/1 -> Sum1/2
  Sum/1 -> Gain18/1, Gain17/1
  Demux/1 -> Transfer Fcn (with initial outputs)3/1
  Demux/2 -> Transfer Fcn (with initial outputs)1/1
  X/1 -> Park/2(abc)
  Gain18/1 -> Sum10/2
  Integrator2/1 -> Sum10/1
  Gain17/1 -> Integrator2/1
  Gain12/1 -> omega_PLL/1
  Demux/3 -> Terminator/1

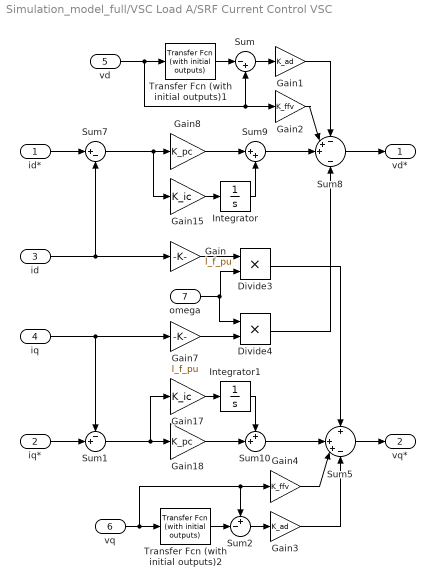
== system Simulation_model_full/VSC Load A/SRF Current Control VSC ==
  id* : Inport
  iq* : Inport  Port=2
  id : Inport  Port=3
  iq : Inport  Port=4
  vd : Inport  Port=5
  vq : Inport  Port=6
  omega : Inport  Port=7
  Divide3 : Product  Inputs=**
  Divide4 : Product  Inputs=**
  Gain : Gain  Gain=l_f_pu
  Gain1 : Gain  Gain=K_ad
  Gain15 : Gain  Gain=K_ic
  Gain17 : Gain  Gain=K_ic
  Gain18 : Gain  Gain=K_pc
  Gain2 : Gain  Gain=K_ffv
  Gain3 : Gain  Gain=K_ad
  Gain4 : Gain  Gain=K_ffv
  Gain7 : Gain  Gain=l_f_pu
  Gain8 : Gain  Gain=K_pc
  Integrator : Integrator  InitialCondition=1
  Integrator1 : Integrator
  Sum : Sum  Inputs=|-+
  Sum1 : Sum  Inputs=-+|
  Sum10 : Sum  Inputs=++|
  Sum2 : Sum  Inputs=+-|
  Sum5 : Sum  Inputs=+|++-
  Sum7 : Sum  Inputs=|+-
  Sum8 : Sum  Inputs=-++|-
  Sum9 : Sum  Inputs=|++
  Transfer Fcn (with initial outputs)1 : simulink_extras/Additional Linear/Transfer Fcn (with initial outputs)  N=[omega_ad]  D="[1  omega_ad]"  Y0=1  U0=1
  Transfer Fcn (with initial outputs)2 : simulink_extras/Additional Linear/Transfer Fcn (with initial outputs)  N=[omega_ad]  D="[1  omega_ad]"  Y0=0  U0=0
  vd* : Outport
  vq* : Outport  Port=2
  wires:
  iq*/1 -> Sum1/2
  Sum7/1 -> Gain15/1, Gain8/1
  Gain15/1 -> Integrator/1
  Sum1/1 -> Gain18/1, Gain17/1
  Divide3/1 -> Sum5/1
  Divide4/1 -> Sum8/4
  Gain7/1 -> Divide4/2
  Gain/1 -> Divide3/1
  Gain17/1 -> Integrator1/1
  Sum9/1 -> Sum8/3
  Integrator1/1 -> Sum10/1
  omega/1 -> Divide4/1, Divide3/2
  Gain18/1 -> Sum10/2
  Sum8/1 -> vd*/1
  Sum10/1 -> Sum5/2
  Gain8/1 -> Sum9/1
  iq/1 -> Gain7/1, Sum1/1
  Integrator/1 -> Sum9/2
  id/1 -> Gain/1, Sum7/2
  id*/1 -> Sum7/1
  Sum5/1 -> vq*/1
  Transfer Fcn (with initial outputs)1/1 -> Sum/1
  Sum/1 -> Gain1/1
  vd/1 -> Transfer Fcn (with initial outputs)1/1, Sum/2, Gain2/1
  Sum2/1 -> Gain3/1
  vq/1 -> Sum2/1, Gain4/1, Transfer Fcn (with initial outputs)2/1
  Transfer Fcn (with initial outputs)2/1 -> Sum2/2
  Gain4/1 -> Sum5/3
  Gain3/1 -> Sum5/4
  Gain2/1 -> Sum8/2
  Gain1/1 -> Sum8/1

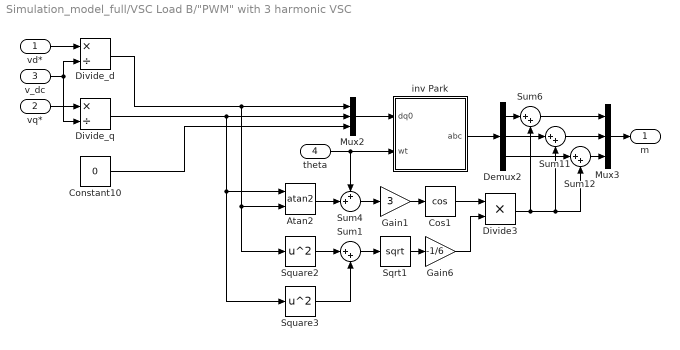
== system Simulation_model_full/VSC Load B/"PWM" with 3 harmonic VSC ==
  vd* : Inport
  vq* : Inport  Port=2
  v_dc : Inport  Port=3
  theta : Inport  Port=4
  Atan2 : Trigonometry  Operator=atan2
  Constant10 : Constant  Value=0
  Cos1 : Trigonometry  Operator=cos
  Demux2 : Demux  Outputs=3
  Divide3 : Product  Inputs=**
  Divide_d : Product  Inputs=*/
  Divide_q : Product  Inputs=*/
  Gain1 : Gain  Gain=3
  Gain6 : Gain  Gain=-1/6
  Mux2 : Mux  Inputs=3
  Mux3 : Mux  Inputs=3
  Sqrt1 : Sqrt  SaturateOnIntegerOverflow=on
  Square2 : Math  Operator=square  SaturateOnIntegerOverflow=on
  Square3 : Math  Operator=square  SaturateOnIntegerOverflow=on
  Sum{1,6,11..12} (4 alike) : Sum  Inputs=|++
  Sum4 : Sum  Inputs=++|
  inv Park : MATLAB Function  TreatAsAtomicUnit=on
  m : Outport
  wires:
  Constant10/1 -> Mux2/3
  Demux2/2 -> Sum11/1
  Sum4/1 -> Gain1/1
  Square2/1 -> Sum1/1
  Demux2/3 -> Sum12/1
  Divide3/1 -> Sum12/2, Sum11/2, Sum6/2
  Atan2/1 -> Sum4/2
  theta/1 -> Sum4/1, inv Park/2(wt)
  Gain6/1 -> Divide3/2
  Gain1/1 -> Cos1/1
  Sum12/1 -> Mux3/3
  Demux2/1 -> Sum6/1
  Sum6/1 -> Mux3/1
  Square3/1 -> Sum1/2
  Sum1/1 -> Sqrt1/1
  Cos1/1 -> Divide3/1
  Sum11/1 -> Mux3/2
  Sqrt1/1 -> Gain6/1
  Mux2/1 -> inv Park/1(dq0)
  vq*/1 -> Divide_q/1
  v_dc/1 -> Divide_d/2, Divide_q/2
  vd*/1 -> Divide_d/1
  Divide_d/1 -> Mux2/1, Atan2/2, Square2/1
  Divide_q/1 -> Square3/1, Atan2/1, Mux2/2
  Mux3/1 -> m/1
  inv Park/1(abc) -> Demux2/1

== system Simulation_model_full/VSC Load B/DC Voltage Control VSC ==
  v_dc* : Inport
  v_dc : Inport  Port=2
  Gain : Gain  Gain=-1
  Gain20 : Gain  Gain=K_idc
  Gain21 : Gain  Gain=K_pdc
  Integrator3 : Integrator
  Sum15 : Sum  Inputs=|++
  Sum16 : Sum  Inputs=|+-
  id* : Outport
  wires:
  Gain21/1 -> Sum15/1
  Sum16/1 -> Gain21/1, Gain20/1
  Integrator3/1 -> Sum15/2
  v_dc*/1 -> Sum16/1
  v_dc/1 -> Sum16/2
  Gain20/1 -> Integrator3/1
  Sum15/1 -> Gain/1
  Gain/1 -> id*/1

== system Simulation_model_full/VSC Load B/PLL VSC ==
  X : Inport
  Atan2 : Trigonometry  Operator=atan2  OutputSignalType=real
  Constant : Constant  Value=0
  Constant1 : Constant  Value=fb
  Demux : Demux  Outputs=3
  Gain : Gain  Gain=K_vco
  Gain12 : Gain  Gain=1/omega_b
  Gain17 : Gain  Gain=K_iPLL
  Gain18 : Gain  Gain=K_pPLL
  Integrator2 : Integrator
  Park : MATLAB Function  TreatAsAtomicUnit=on
  Sum : Sum  Inputs=|++
  Sum1 : Sum  Inputs=++|
  Sum10 : Sum  Inputs=++|
  Terminator : Terminator
  Transfer Fcn (with initial outputs)1 : simulink_extras/Additional Linear/Transfer Fcn (with initial outputs)  N=[1]  D=[T_fPLL, 1]  Y0=0  U0=0
  Transfer Fcn (with initial outputs)3 : simulink_extras/Additional Linear/Transfer Fcn (with initial outputs)  N=[1]  D=[T_fPLL, 1]  Y0=1  U0=1
  VCO : Integrator  WrapState=on  WrappedStateUpperValue=2*pi  WrappedStateLowerValue=0
  theta_PLL : Outport
  omega_PLL : Outport  Port=2
  wires:
  Transfer Fcn (with initial outputs)1/1 -> Atan2/1
  Transfer Fcn (with initial outputs)3/1 -> Atan2/2
  Constant/1 -> Sum/1
  VCO/1 -> theta_PLL/1, Park/1(wt)
  Sum1/1 -> Gain/1
  Gain/1 -> Gain12/1, VCO/1
  Constant1/1 -> Sum1/1
  Park/1(dq0) -> Demux/1
  Atan2/1 -> Sum/2
  Sum10/1 -> Sum1/2
  Sum/1 -> Gain18/1, Gain17/1
  Demux/1 -> Transfer Fcn (with initial outputs)3/1
  Demux/2 -> Transfer Fcn (with initial outputs)1/1
  X/1 -> Park/2(abc)
  Gain18/1 -> Sum10/2
  Integrator2/1 -> Sum10/1
  Gain17/1 -> Integrator2/1
  Gain12/1 -> omega_PLL/1
  Demux/3 -> Terminator/1

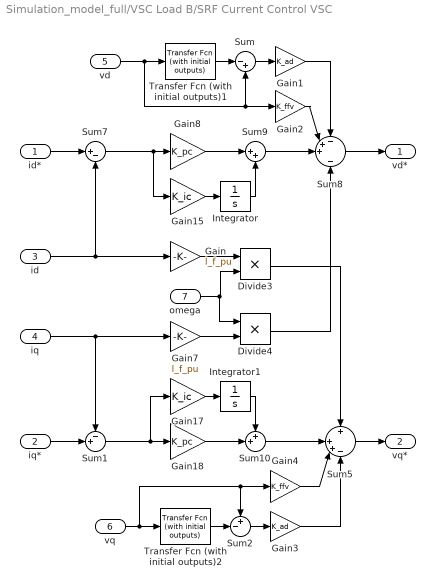
== system Simulation_model_full/VSC Load B/SRF Current Control VSC ==
  id* : Inport
  iq* : Inport  Port=2
  id : Inport  Port=3
  iq : Inport  Port=4
  vd : Inport  Port=5
  vq : Inport  Port=6
  omega : Inport  Port=7
  Divide3 : Product  Inputs=**
  Divide4 : Product  Inputs=**
  Gain : Gain  Gain=l_f_pu
  Gain1 : Gain  Gain=K_ad
  Gain15 : Gain  Gain=K_ic
  Gain17 : Gain  Gain=K_ic
  Gain18 : Gain  Gain=K_pc
  Gain2 : Gain  Gain=K_ffv
  Gain3 : Gain  Gain=K_ad
  Gain4 : Gain  Gain=K_ffv
  Gain7 : Gain  Gain=l_f_pu
  Gain8 : Gain  Gain=K_pc
  Integrator : Integrator  InitialCondition=1
  Integrator1 : Integrator
  Sum : Sum  Inputs=|-+
  Sum1 : Sum  Inputs=-+|
  Sum10 : Sum  Inputs=++|
  Sum2 : Sum  Inputs=+-|
  Sum5 : Sum  Inputs=+|++-
  Sum7 : Sum  Inputs=|+-
  Sum8 : Sum  Inputs=-++|-
  Sum9 : Sum  Inputs=|++
  Transfer Fcn (with initial outputs)1 : simulink_extras/Additional Linear/Transfer Fcn (with initial outputs)  N=[omega_ad]  D="[1  omega_ad]"  Y0=1  U0=1
  Transfer Fcn (with initial outputs)2 : simulink_extras/Additional Linear/Transfer Fcn (with initial outputs)  N=[omega_ad]  D="[1  omega_ad]"  Y0=0  U0=0
  vd* : Outport
  vq* : Outport  Port=2
  wires:
  iq*/1 -> Sum1/2
  Sum7/1 -> Gain15/1, Gain8/1
  Gain15/1 -> Integrator/1
  Sum1/1 -> Gain18/1, Gain17/1
  Divide3/1 -> Sum5/1
  Divide4/1 -> Sum8/4
  Gain7/1 -> Divide4/2
  Gain/1 -> Divide3/1
  Gain17/1 -> Integrator1/1
  Sum9/1 -> Sum8/3
  Integrator1/1 -> Sum10/1
  omega/1 -> Divide4/1, Divide3/2
  Gain18/1 -> Sum10/2
  Sum8/1 -> vd*/1
  Sum10/1 -> Sum5/2
  Gain8/1 -> Sum9/1
  iq/1 -> Gain7/1, Sum1/1
  Integrator/1 -> Sum9/2
  id/1 -> Gain/1, Sum7/2
  id*/1 -> Sum7/1
  Sum5/1 -> vq*/1
  Transfer Fcn (with initial outputs)1/1 -> Sum/1
  Sum/1 -> Gain1/1
  vd/1 -> Transfer Fcn (with initial outputs)1/1, Sum/2, Gain2/1
  Sum2/1 -> Gain3/1
  vq/1 -> Sum2/1, Gain4/1, Transfer Fcn (with initial outputs)2/1
  Transfer Fcn (with initial outputs)2/1 -> Sum2/2
  Gain4/1 -> Sum5/3
  Gain3/1 -> Sum5/4
  Gain2/1 -> Sum8/2
  Gain1/1 -> Sum8/1

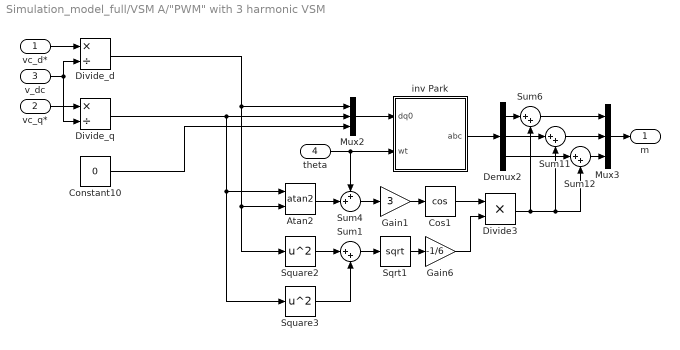
== system Simulation_model_full/VSM A/"PWM" with 3 harmonic VSM ==
  vc_d* : Inport
  vc_q* : Inport  Port=2
  v_dc : Inport  Port=3
  theta : Inport  Port=4
  Atan2 : Trigonometry  Operator=atan2
  Constant10 : Constant  Value=0
  Cos1 : Trigonometry  Operator=cos
  Demux2 : Demux  Outputs=3
  Divide3 : Product  Inputs=**
  Divide_d : Product  Inputs=*/
  Divide_q : Product  Inputs=*/
  Gain1 : Gain  Gain=3
  Gain6 : Gain  Gain=-1/6
  Mux2 : Mux  Inputs=3
  Mux3 : Mux  Inputs=3
  Sqrt1 : Sqrt  SaturateOnIntegerOverflow=on
  Square2 : Math  Operator=square  SaturateOnIntegerOverflow=on
  Square3 : Math  Operator=square  SaturateOnIntegerOverflow=on
  Sum{1,6,11..12} (4 alike) : Sum  Inputs=|++
  Sum4 : Sum  Inputs=++|
  inv Park : MATLAB Function  TreatAsAtomicUnit=on
  m : Outport
  wires:
  Constant10/1 -> Mux2/3
  Demux2/2 -> Sum11/1
  Sum4/1 -> Gain1/1
  Square2/1 -> Sum1/1
  Demux2/3 -> Sum12/1
  Divide3/1 -> Sum12/2, Sum11/2, Sum6/2
  Atan2/1 -> Sum4/2
  theta/1 -> Sum4/1, inv Park/2(wt)
  Gain6/1 -> Divide3/2
  Gain1/1 -> Cos1/1
  Sum12/1 -> Mux3/3
  Demux2/1 -> Sum6/1
  Sum6/1 -> Mux3/1
  Square3/1 -> Sum1/2
  Sum1/1 -> Sqrt1/1
  Cos1/1 -> Divide3/1
  Sum11/1 -> Mux3/2
  Sqrt1/1 -> Gain6/1
  Mux2/1 -> inv Park/1(dq0)
  vc_q*/1 -> Divide_q/1
  v_dc/1 -> Divide_d/2, Divide_q/2
  vc_d*/1 -> Divide_d/1
  Mux3/1 -> m/1
  inv Park/1(abc) -> Demux2/1
  Divide_d/1 -> Mux2/1, Atan2/2, Square2/1
  Divide_q/1 -> Square3/1, Atan2/1, Mux2/2

== system Simulation_model_full/VSM A/Frequency Control (Governor) VSM ==
  p* : Inport
  omega* VMS : Inport  Port=2
  omega VMS : Inport  Port=3
  Gain8 : Gain  Gain=K_omega
  Sum : Sum  Inputs=++|
  Sum1 : Sum  Inputs=|+-
  pr* : Outport
  wires:
  Sum/1 -> pr*/1
  omega* VMS/1 -> Sum1/1
  omega VMS/1 -> Sum1/2
  p*/1 -> Sum/1
  Sum1/1 -> Gain8/1
  Gain8/1 -> Sum/2

== system Simulation_model_full/VSM A/Inertia Model VSM ==
  p : Inport
  pr* : Inport  Port=2
  triger : Inport  Port=3
  omega_PLL : Inport  Port=4
  theta_PLL : Inport  Port=5
  Gain : Gain  Gain=1/Ta
  Gain1 : Gain  Gain=omega_b
  Gain3 : Gain  Gain=Kd
  Integrator1 : Integrator  ExternalReset=level hold  InitialConditionSource=external  InitialCondition=1  WrapState=on  WrappedStateUpperValue=2*pi  WrappedStateLowerValue=0
  Integrator2 : Integrator  ExternalReset=level hold  InitialConditionSource=external  InitialCondition=1
  Sum : Sum  Inputs=-+|
  Sum1 : Sum  Inputs=-+-
  Transfer Fcn (with initial outputs) : simulink_extras/Additional Linear/Transfer Fcn (with initial outputs)  Commented=on  N=[omega_d]  D="[1  omega_d]"  Y0=1  U0=1
  omega_VSM : Outport
  theta_VSM : Outport  Port=2
  wires:
  Gain/1 -> Integrator2/1
  Gain3/1 -> Sum1/3
  Sum1/1 -> Gain/1
  p/1 -> Sum1/1
  pr*/1 -> Sum1/2
  Integrator1/1 -> theta_VSM/1
  Integrator2/1 -> Sum/2, Transfer Fcn (with initial outputs)/1, Gain1/1, omega_VSM/1
  theta_PLL/1 -> Integrator1/3
  triger/1 -> Integrator2/2, Integrator1/2
  Gain1/1 -> Integrator1/1
  omega_PLL/1 -> Integrator2/3, Sum/1
  Sum/1 -> Gain3/1

== system Simulation_model_full/VSM A/PLL Vf VSM ==
  Vo : Inport
  Atan2 : Trigonometry  Operator=atan2  OutputSignalType=real
  Constant1 : Constant  Value=fb
  Demux : Demux  Outputs=3
  Gain : Gain  Gain=K_vco
  Gain12 : Gain  Gain=1/omega_b
  Gain17 : Gain  Gain=K_iPLL
  Gain18 : Gain  Gain=K_pPLL
  Integrator2 : Integrator
  Park : MATLAB Function  TreatAsAtomicUnit=on
  Sum1 : Sum  Inputs=++|
  Sum10 : Sum  Inputs=++|
  Terminator : Terminator
  Transfer Fcn (with initial outputs)1 : simulink_extras/Additional Linear/Transfer Fcn (with initial outputs)  N=[1]  D=[T_fPLL, 1]  Y0=0  U0=0
  Transfer Fcn (with initial outputs)3 : simulink_extras/Additional Linear/Transfer Fcn (with initial outputs)  N=[1]  D=[T_fPLL, 1]  Y0=1  U0=1
  VCO : Integrator  WrapState=on  WrappedStateUpperValue=2*pi  WrappedStateLowerValue=0
  theta_PLL : Outport
  omega_PLL : Outport  Port=2
  wires:
  Transfer Fcn (with initial outputs)1/1 -> Atan2/1
  Transfer Fcn (with initial outputs)3/1 -> Atan2/2
  VCO/1 -> theta_PLL/1, Park/1(theta)
  Sum1/1 -> Gain/1
  Gain/1 -> Gain12/1, VCO/1
  Constant1/1 -> Sum1/1
  Park/1(dq0) -> Demux/1
  Sum10/1 -> Sum1/2
  Atan2/1 -> Gain18/1, Gain17/1
  Demux/1 -> Transfer Fcn (with initial outputs)3/1
  Demux/2 -> Transfer Fcn (with initial outputs)1/1
  Vo/1 -> Park/2(abc)
  Gain18/1 -> Sum10/2
  Integrator2/1 -> Sum10/1
  Gain17/1 -> Integrator2/1
  Gain12/1 -> omega_PLL/1
  Demux/3 -> Terminator/1

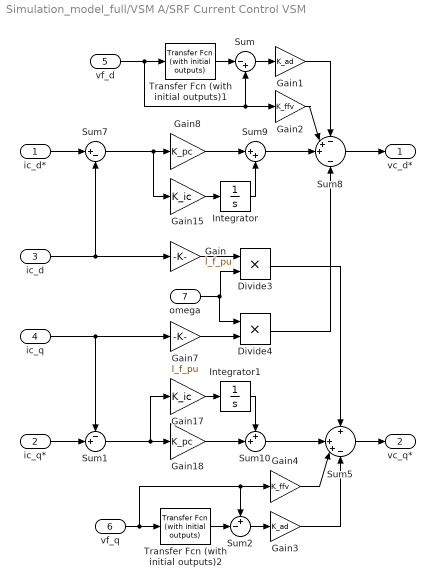
== system Simulation_model_full/VSM A/SRF Current Control VSM ==
  ic_d* : Inport
  ic_q* : Inport  Port=2
  ic_d : Inport  Port=3
  ic_q : Inport  Port=4
  vf_d : Inport  Port=5
  vf_q : Inport  Port=6
  omega : Inport  Port=7
  Divide3 : Product  Inputs=**
  Divide4 : Product  Inputs=**
  Gain : Gain  Gain=l_f_pu
  Gain1 : Gain  Gain=K_ad
  Gain15 : Gain  Gain=K_ic
  Gain17 : Gain  Gain=K_ic
  Gain18 : Gain  Gain=K_pc
  Gain2 : Gain  Gain=K_ffv
  Gain3 : Gain  Gain=K_ad
  Gain4 : Gain  Gain=K_ffv
  Gain7 : Gain  Gain=l_f_pu
  Gain8 : Gain  Gain=K_pc
  Integrator : Integrator  InitialCondition=1
  Integrator1 : Integrator
  Sum : Sum  Inputs=|-+
  Sum1 : Sum  Inputs=-+|
  Sum10 : Sum  Inputs=++|
  Sum2 : Sum  Inputs=+-|
  Sum5 : Sum  Inputs=+|++-
  Sum7 : Sum  Inputs=|+-
  Sum8 : Sum  Inputs=-++|-
  Sum9 : Sum  Inputs=|++
  Transfer Fcn (with initial outputs)1 : simulink_extras/Additional Linear/Transfer Fcn (with initial outputs)  N=[omega_ad]  D="[1  omega_ad]"  Y0=1  U0=1
  Transfer Fcn (with initial outputs)2 : simulink_extras/Additional Linear/Transfer Fcn (with initial outputs)  N=[omega_ad]  D="[1  omega_ad]"  Y0=0  U0=0
  vc_d* : Outport
  vc_q* : Outport  Port=2
  wires:
  ic_q*/1 -> Sum1/2
  Sum7/1 -> Gain15/1, Gain8/1
  Gain15/1 -> Integrator/1
  Sum1/1 -> Gain18/1, Gain17/1
  Divide3/1 -> Sum5/1
  Divide4/1 -> Sum8/4
  Gain7/1 -> Divide4/2
  Gain/1 -> Divide3/1
  Gain17/1 -> Integrator1/1
  Sum9/1 -> Sum8/3
  Integrator1/1 -> Sum10/1
  omega/1 -> Divide4/1, Divide3/2
  Gain18/1 -> Sum10/2
  Sum8/1 -> vc_d*/1
  Sum10/1 -> Sum5/2
  Gain8/1 -> Sum9/1
  ic_q/1 -> Gain7/1, Sum1/1
  Integrator/1 -> Sum9/2
  ic_d/1 -> Gain/1, Sum7/2
  ic_d*/1 -> Sum7/1
  Sum5/1 -> vc_q*/1
  Transfer Fcn (with initial outputs)1/1 -> Sum/1
  Sum/1 -> Gain1/1
  Gain1/1 -> Sum8/1
  vf_d/1 -> Transfer Fcn (with initial outputs)1/1, Sum/2, Gain2/1
  Gain2/1 -> Sum8/2
  Sum2/1 -> Gain3/1
  vf_q/1 -> Sum2/1, Gain4/1, Transfer Fcn (with initial outputs)2/1
  Transfer Fcn (with initial outputs)2/1 -> Sum2/2
  Gain4/1 -> Sum5/3
  Gain3/1 -> Sum5/4

== system Simulation_model_full/VSM A/Voltage Control (AVR) VSM ==
  vhat* : Inport
  vhat_f : Inport  Port=2
  q* : Inport  Port=3
  q : Inport  Port=4
  triger : Inport  Port=5
  Gain15 : Gain  Gain=K_iv
  Gain2 : Gain  Gain=Kq
  Gain8 : Gain  Gain=K_pv
  Integrator : Integrator  ExternalReset=level hold
  Sum1 : Sum  Inputs=-++
  Sum2 : Sum  Inputs=|+-
  Sum9 : Sum  Inputs=|++
  Transfer Fcn (with initial outputs) : simulink_extras/Additional Linear/Transfer Fcn (with initial outputs)  N=[omega_qf]  D="[1  omega_qf]"  Y0=0  U0=0
  vhat_e : Outport
  wires:
  Sum9/1 -> vhat_e/1
  Integrator/1 -> Sum9/2
  Sum1/1 -> Gain15/1, Gain8/1
  Gain15/1 -> Integrator/1
  Gain8/1 -> Sum9/1
  vhat_f/1 -> Sum1/1
  q*/1 -> Sum2/1
  q/1 -> Transfer Fcn (with initial outputs)/1
  Transfer Fcn (with initial outputs)/1 -> Sum2/2
  Sum2/1 -> Gain2/1
  vhat*/1 -> Sum1/2
  Gain2/1 -> Sum1/3
  triger/1 -> Integrator/2

== system Simulation_model_full/VSM A1/"PWM" with 3 harmonic VSM ==
  vc_d* : Inport
  vc_q* : Inport  Port=2
  v_dc : Inport  Port=3
  theta : Inport  Port=4
  Atan2 : Trigonometry  Operator=atan2
  Constant10 : Constant  Value=0
  Cos1 : Trigonometry  Operator=cos
  Demux2 : Demux  Outputs=3
  Divide3 : Product  Inputs=**
  Divide_d : Product  Inputs=*/
  Divide_q : Product  Inputs=*/
  Gain1 : Gain  Gain=3
  Gain6 : Gain  Gain=-1/6
  Mux2 : Mux  Inputs=3
  Mux3 : Mux  Inputs=3
  Sqrt1 : Sqrt  SaturateOnIntegerOverflow=on
  Square2 : Math  Operator=square  SaturateOnIntegerOverflow=on
  Square3 : Math  Operator=square  SaturateOnIntegerOverflow=on
  Sum{1,6,11..12} (4 alike) : Sum  Inputs=|++
  Sum4 : Sum  Inputs=++|
  inv Park : MATLAB Function  TreatAsAtomicUnit=on
  m : Outport
  wires:
  Constant10/1 -> Mux2/3
  Demux2/2 -> Sum11/1
  Sum4/1 -> Gain1/1
  Square2/1 -> Sum1/1
  Demux2/3 -> Sum12/1
  Divide3/1 -> Sum12/2, Sum11/2, Sum6/2
  Atan2/1 -> Sum4/2
  theta/1 -> Sum4/1, inv Park/2(wt)
  Gain6/1 -> Divide3/2
  Gain1/1 -> Cos1/1
  Sum12/1 -> Mux3/3
  Demux2/1 -> Sum6/1
  Sum6/1 -> Mux3/1
  Square3/1 -> Sum1/2
  Sum1/1 -> Sqrt1/1
  Cos1/1 -> Divide3/1
  Sum11/1 -> Mux3/2
  Sqrt1/1 -> Gain6/1
  Mux2/1 -> inv Park/1(dq0)
  vc_q*/1 -> Divide_q/1
  v_dc/1 -> Divide_d/2, Divide_q/2
  vc_d*/1 -> Divide_d/1
  Mux3/1 -> m/1
  inv Park/1(abc) -> Demux2/1
  Divide_d/1 -> Mux2/1, Atan2/2, Square2/1
  Divide_q/1 -> Square3/1, Atan2/1, Mux2/2

== system Simulation_model_full/VSM A1/Frequency Control (Governor) VSM ==
  p* : Inport
  omega* VMS : Inport  Port=2
  omega VMS : Inport  Port=3
  Gain8 : Gain  Gain=K_omega
  Sum : Sum  Inputs=++|
  Sum1 : Sum  Inputs=|+-
  pr* : Outport
  wires:
  Sum/1 -> pr*/1
  omega* VMS/1 -> Sum1/1
  omega VMS/1 -> Sum1/2
  p*/1 -> Sum/1
  Sum1/1 -> Gain8/1
  Gain8/1 -> Sum/2

== system Simulation_model_full/VSM A1/Inertia Model VSM ==
  p : Inport
  pr* : Inport  Port=2
  triger : Inport  Port=3
  omega_PLL : Inport  Port=4
  theta_PLL : Inport  Port=5
  Gain : Gain  Gain=1/Ta
  Gain1 : Gain  Gain=omega_b
  Gain3 : Gain  Gain=Kd
  Integrator1 : Integrator  ExternalReset=level hold  InitialConditionSource=external  InitialCondition=1  WrapState=on  WrappedStateUpperValue=2*pi  WrappedStateLowerValue=0
  Integrator2 : Integrator  ExternalReset=level hold  InitialConditionSource=external  InitialCondition=1
  Sum : Sum  Inputs=-+|
  Sum1 : Sum  Inputs=-+-
  Transfer Fcn (with initial outputs) : simulink_extras/Additional Linear/Transfer Fcn (with initial outputs)  Commented=on  N=[omega_d]  D="[1  omega_d]"  Y0=1  U0=1
  omega_VSM : Outport
  theta_VSM : Outport  Port=2
  wires:
  Gain/1 -> Integrator2/1
  Gain3/1 -> Sum1/3
  Sum1/1 -> Gain/1
  p/1 -> Sum1/1
  pr*/1 -> Sum1/2
  Integrator1/1 -> theta_VSM/1
  Integrator2/1 -> Sum/2, Transfer Fcn (with initial outputs)/1, Gain1/1, omega_VSM/1
  theta_PLL/1 -> Integrator1/3
  triger/1 -> Integrator2/2, Integrator1/2
  Gain1/1 -> Integrator1/1
  omega_PLL/1 -> Integrator2/3, Sum/1
  Sum/1 -> Gain3/1

== system Simulation_model_full/VSM A1/PLL Vf VSM ==
  Vo : Inport
  Atan2 : Trigonometry  Operator=atan2  OutputSignalType=real
  Constant1 : Constant  Value=fb
  Demux : Demux  Outputs=3
  Gain : Gain  Gain=K_vco
  Gain12 : Gain  Gain=1/omega_b
  Gain17 : Gain  Gain=K_iPLL
  Gain18 : Gain  Gain=K_pPLL
  Integrator2 : Integrator
  Park : MATLAB Function  TreatAsAtomicUnit=on
  Sum1 : Sum  Inputs=++|
  Sum10 : Sum  Inputs=++|
  Terminator : Terminator
  Transfer Fcn (with initial outputs)1 : simulink_extras/Additional Linear/Transfer Fcn (with initial outputs)  N=[1]  D=[T_fPLL, 1]  Y0=0  U0=0
  Transfer Fcn (with initial outputs)3 : simulink_extras/Additional Linear/Transfer Fcn (with initial outputs)  N=[1]  D=[T_fPLL, 1]  Y0=1  U0=1
  VCO : Integrator  WrapState=on  WrappedStateUpperValue=2*pi  WrappedStateLowerValue=0
  theta_PLL : Outport
  omega_PLL : Outport  Port=2
  wires:
  Transfer Fcn (with initial outputs)1/1 -> Atan2/1
  Transfer Fcn (with initial outputs)3/1 -> Atan2/2
  VCO/1 -> theta_PLL/1, Park/1(theta)
  Sum1/1 -> Gain/1
  Gain/1 -> Gain12/1, VCO/1
  Constant1/1 -> Sum1/1
  Park/1(dq0) -> Demux/1
  Sum10/1 -> Sum1/2
  Atan2/1 -> Gain18/1, Gain17/1
  Demux/1 -> Transfer Fcn (with initial outputs)3/1
  Demux/2 -> Transfer Fcn (with initial outputs)1/1
  Vo/1 -> Park/2(abc)
  Gain18/1 -> Sum10/2
  Integrator2/1 -> Sum10/1
  Gain17/1 -> Integrator2/1
  Gain12/1 -> omega_PLL/1
  Demux/3 -> Terminator/1
